simulink model "RAM_Design"  (R2025a)
settings: Solver=FixedStepDiscrete  StartTime=0.0  StopTime=10  FixedStep=1e-6  RelTol=1e-3
undefined symbols (not defined in the file): Bit_1, Bit_2, Bit_3, Bit_4, Bit_5, Bit_6, Bit_7, Bit_8
libraries: fl_lib x320, nesl_utility x136, simulink_extras x57
(part 3 of 5)

== system RAM_Design/Subsystem1/8Bit RAM 63/Subsystem13 ==
  Enable : Inport
  Data : Inport  Port=2
  Store : Inport  Port=3
  AND : Logic  IconShape=distinctive  AllPortsSameDT=off  OutDataTypeStr=boolean
  Cast To Double : DataTypeConversion  OutDataTypeStr=double  SaturateOnIntegerOverflow=off  RndMeth=Floor
  Controlled Voltage Source : fl_lib/Electrical/Electrical Sources/Controlled Voltage Source
  D Latch : simulink_extras/Flip Flops/D Latch
  Delay One Step : Delay  DelayLength=1
  Electrical Reference : fl_lib/Electrical/Electrical Elements/Electrical Reference
  Gain : Gain  Gain=5
  Simulink-PS Converter : nesl_utility/Simulink-PS Converter  PhysicalDomain=network_engine_domain  SubClassName=ps_input  LeftPortType=input  RightPortType=output  PseudoPeriodic=off  Frequencies=[]  NoiseDistribution=none  NoiseParameters=[]  Unit=1  AffineConversion=off  FilteringAndDerivatives=provide  SimscapeFilterOrder=1  InputFilterTimeConstant=0.001  UdotUserProvided=0
  Q : PMIOPort  Side=Right
  StoredVal : Outport
  wires:
  AND/1 -> Delay One Step/1
  Store/1 -> D Latch/2
  Gain/1 -> Simulink-PS Converter/1
  D Latch/1 -> StoredVal/1, AND/1
  Cast To Double/1 -> Gain/1
  Enable/1 -> AND/2
  Data/1 -> D Latch/1
  Delay One Step/1 -> Cast To Double/1
  connections:
  Controlled Voltage Source/RConn1 -- Simulink-PS Converter/RConn1
  Electrical Reference/LConn1 -- Controlled Voltage Source/RConn2
  Controlled Voltage Source/LConn1 -- Q/RConn1

== system RAM_Design/Subsystem1/8Bit RAM 63/Subsystem14 ==
  Enable : Inport
  Data : Inport  Port=2
  Store : Inport  Port=3
  AND : Logic  IconShape=distinctive  AllPortsSameDT=off  OutDataTypeStr=boolean
  Cast To Double : DataTypeConversion  OutDataTypeStr=double  SaturateOnIntegerOverflow=off  RndMeth=Floor
  Controlled Voltage Source : fl_lib/Electrical/Electrical Sources/Controlled Voltage Source
  D Latch : simulink_extras/Flip Flops/D Latch
  Delay One Step : Delay  DelayLength=1
  Electrical Reference : fl_lib/Electrical/Electrical Elements/Electrical Reference
  Gain : Gain  Gain=5
  Simulink-PS Converter : nesl_utility/Simulink-PS Converter  PhysicalDomain=network_engine_domain  SubClassName=ps_input  LeftPortType=input  RightPortType=output  PseudoPeriodic=off  Frequencies=[]  NoiseDistribution=none  NoiseParameters=[]  Unit=1  AffineConversion=off  FilteringAndDerivatives=provide  SimscapeFilterOrder=1  InputFilterTimeConstant=0.001  UdotUserProvided=0
  Q : PMIOPort  Side=Right
  StoredVal : Outport
  wires:
  AND/1 -> Delay One Step/1
  Store/1 -> D Latch/2
  Gain/1 -> Simulink-PS Converter/1
  D Latch/1 -> StoredVal/1, AND/1
  Cast To Double/1 -> Gain/1
  Enable/1 -> AND/2
  Data/1 -> D Latch/1
  Delay One Step/1 -> Cast To Double/1
  connections:
  Controlled Voltage Source/RConn1 -- Simulink-PS Converter/RConn1
  Electrical Reference/LConn1 -- Controlled Voltage Source/RConn2
  Controlled Voltage Source/LConn1 -- Q/RConn1

== system RAM_Design/Subsystem1/8Bit RAM 63/Subsystem15 ==
  Enable : Inport
  Data : Inport  Port=2
  Store : Inport  Port=3
  AND : Logic  IconShape=distinctive  AllPortsSameDT=off  OutDataTypeStr=boolean
  Cast To Double : DataTypeConversion  OutDataTypeStr=double  SaturateOnIntegerOverflow=off  RndMeth=Floor
  Controlled Voltage Source : fl_lib/Electrical/Electrical Sources/Controlled Voltage Source
  D Latch : simulink_extras/Flip Flops/D Latch
  Delay One Step : Delay  DelayLength=1
  Electrical Reference : fl_lib/Electrical/Electrical Elements/Electrical Reference
  Gain : Gain  Gain=5
  Simulink-PS Converter : nesl_utility/Simulink-PS Converter  PhysicalDomain=network_engine_domain  SubClassName=ps_input  LeftPortType=input  RightPortType=output  PseudoPeriodic=off  Frequencies=[]  NoiseDistribution=none  NoiseParameters=[]  Unit=1  AffineConversion=off  FilteringAndDerivatives=provide  SimscapeFilterOrder=1  InputFilterTimeConstant=0.001  UdotUserProvided=0
  Q : PMIOPort  Side=Right
  StoredVal : Outport
  wires:
  AND/1 -> Delay One Step/1
  Store/1 -> D Latch/2
  Gain/1 -> Simulink-PS Converter/1
  D Latch/1 -> StoredVal/1, AND/1
  Cast To Double/1 -> Gain/1
  Enable/1 -> AND/2
  Data/1 -> D Latch/1
  Delay One Step/1 -> Cast To Double/1
  connections:
  Controlled Voltage Source/RConn1 -- Simulink-PS Converter/RConn1
  Electrical Reference/LConn1 -- Controlled Voltage Source/RConn2
  Controlled Voltage Source/LConn1 -- Q/RConn1

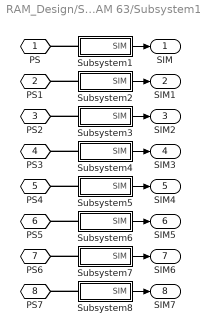
== system RAM_Design/Subsystem1/8Bit RAM 63/Subsystem16 ==
  Subsystem1 : Subsystem
  Subsystem2 : Subsystem
  Subsystem3 : Subsystem
  Subsystem4 : Subsystem
  Subsystem5 : Subsystem
  Subsystem6 : Subsystem
  Subsystem7 : Subsystem
  Subsystem8 : Subsystem
  PS : PMIOPort  Side=Left
  PS1 : PMIOPort  Port=2  Side=Left
  PS2 : PMIOPort  Port=3  Side=Left
  PS3 : PMIOPort  Port=4  Side=Left
  PS4 : PMIOPort  Port=5  Side=Left
  PS5 : PMIOPort  Port=6  Side=Left
  PS6 : PMIOPort  Port=7  Side=Left
  PS7 : PMIOPort  Port=8  Side=Left
  SIM : Outport
  SIM1 : Outport  Port=2
  SIM2 : Outport  Port=3
  SIM3 : Outport  Port=4
  SIM4 : Outport  Port=5
  SIM5 : Outport  Port=6
  SIM6 : Outport  Port=7
  SIM7 : Outport  Port=8
  wires:
  Subsystem7/1(SIM) -> SIM6/1
  Subsystem8/1(SIM) -> SIM7/1
  Subsystem3/1(SIM) -> SIM2/1
  Subsystem4/1(SIM) -> SIM3/1
  Subsystem6/1(SIM) -> SIM5/1
  Subsystem2/1(SIM) -> SIM1/1
  Subsystem5/1(SIM) -> SIM4/1
  Subsystem1/1(SIM) -> SIM/1
  connections:
  Subsystem1/LConn1 -- PS/RConn1
  Subsystem8/LConn1 -- PS7/RConn1
  Subsystem5/LConn1 -- PS4/RConn1
  Subsystem6/LConn1 -- PS5/RConn1
  Subsystem7/LConn1 -- PS6/RConn1
  Subsystem3/LConn1 -- PS2/RConn1
  Subsystem4/LConn1 -- PS3/RConn1
  Subsystem2/LConn1 -- PS1/RConn1

== system RAM_Design/Subsystem1/8Bit RAM 63/Subsystem2 ==
  Cast To Boolean : DataTypeConversion  OutDataTypeStr=boolean  SaturateOnIntegerOverflow=off  RndMeth=Floor
  Delay One Step : Delay  DelayLength=1
  Electrical Reference : fl_lib/Electrical/Electrical Elements/Electrical Reference
  Gain : Gain  Gain=0.2
  PS-Simulink Converter : nesl_utility/PS-Simulink Converter  PhysicalDomain=network_engine_domain  SubClassName=ps_output  LeftPortType=input  RightPortType=output  PseudoPeriodic=off  Frequencies=[]  VectorFormat=inherit  Unit=inherit  AffineConversion=off
  Voltage Sensor : fl_lib/Electrical/Electrical Sensors/Voltage Sensor
  PS : PMIOPort  Side=Left
  SIM : Outport
  wires:
  PS-Simulink Converter/1 -> Gain/1
  Cast To Boolean/1 -> Delay One Step/1
  Gain/1 -> Cast To Boolean/1
  Delay One Step/1 -> SIM/1
  connections:
  PS/RConn1 -- Voltage Sensor/LConn1
  Electrical Reference/LConn1 -- Voltage Sensor/RConn2
  PS-Simulink Converter/LConn1 -- Voltage Sensor/RConn1

== system RAM_Design/Subsystem1/8Bit RAM 63/Subsystem3 ==
  Cast To Boolean : DataTypeConversion  OutDataTypeStr=boolean  SaturateOnIntegerOverflow=off  RndMeth=Floor
  Delay One Step : Delay  DelayLength=1
  Electrical Reference : fl_lib/Electrical/Electrical Elements/Electrical Reference
  Gain : Gain  Gain=0.2
  PS-Simulink Converter : nesl_utility/PS-Simulink Converter  PhysicalDomain=network_engine_domain  SubClassName=ps_output  LeftPortType=input  RightPortType=output  PseudoPeriodic=off  Frequencies=[]  VectorFormat=inherit  Unit=inherit  AffineConversion=off
  Voltage Sensor : fl_lib/Electrical/Electrical Sensors/Voltage Sensor
  PS : PMIOPort  Side=Left
  SIM : Outport
  wires:
  PS-Simulink Converter/1 -> Gain/1
  Cast To Boolean/1 -> Delay One Step/1
  Gain/1 -> Cast To Boolean/1
  Delay One Step/1 -> SIM/1
  connections:
  PS/RConn1 -- Voltage Sensor/LConn1
  Electrical Reference/LConn1 -- Voltage Sensor/RConn2
  PS-Simulink Converter/LConn1 -- Voltage Sensor/RConn1

== system RAM_Design/Subsystem1/8Bit RAM 63/Subsystem4 ==
  Cast To Boolean : DataTypeConversion  OutDataTypeStr=boolean  SaturateOnIntegerOverflow=off  RndMeth=Floor
  Delay One Step : Delay  DelayLength=1
  Electrical Reference : fl_lib/Electrical/Electrical Elements/Electrical Reference
  Gain : Gain  Gain=0.2
  PS-Simulink Converter : nesl_utility/PS-Simulink Converter  PhysicalDomain=network_engine_domain  SubClassName=ps_output  LeftPortType=input  RightPortType=output  PseudoPeriodic=off  Frequencies=[]  VectorFormat=inherit  Unit=inherit  AffineConversion=off
  Voltage Sensor : fl_lib/Electrical/Electrical Sensors/Voltage Sensor
  PS : PMIOPort  Side=Left
  SIM : Outport
  wires:
  PS-Simulink Converter/1 -> Gain/1
  Cast To Boolean/1 -> Delay One Step/1
  Gain/1 -> Cast To Boolean/1
  Delay One Step/1 -> SIM/1
  connections:
  PS/RConn1 -- Voltage Sensor/LConn1
  Electrical Reference/LConn1 -- Voltage Sensor/RConn2
  PS-Simulink Converter/LConn1 -- Voltage Sensor/RConn1

== system RAM_Design/Subsystem1/8Bit RAM 63/Subsystem5 ==
  Cast To Boolean : DataTypeConversion  OutDataTypeStr=boolean  SaturateOnIntegerOverflow=off  RndMeth=Floor
  Delay One Step : Delay  DelayLength=1
  Electrical Reference : fl_lib/Electrical/Electrical Elements/Electrical Reference
  Gain : Gain  Gain=0.2
  PS-Simulink Converter : nesl_utility/PS-Simulink Converter  PhysicalDomain=network_engine_domain  SubClassName=ps_output  LeftPortType=input  RightPortType=output  PseudoPeriodic=off  Frequencies=[]  VectorFormat=inherit  Unit=inherit  AffineConversion=off
  Voltage Sensor : fl_lib/Electrical/Electrical Sensors/Voltage Sensor
  PS : PMIOPort  Side=Left
  SIM : Outport
  wires:
  PS-Simulink Converter/1 -> Gain/1
  Cast To Boolean/1 -> Delay One Step/1
  Gain/1 -> Cast To Boolean/1
  Delay One Step/1 -> SIM/1
  connections:
  PS/RConn1 -- Voltage Sensor/LConn1
  Electrical Reference/LConn1 -- Voltage Sensor/RConn2
  PS-Simulink Converter/LConn1 -- Voltage Sensor/RConn1

== system RAM_Design/Subsystem1/8Bit RAM 63/Subsystem6 ==
  Cast To Boolean : DataTypeConversion  OutDataTypeStr=boolean  SaturateOnIntegerOverflow=off  RndMeth=Floor
  Delay One Step : Delay  DelayLength=1
  Electrical Reference : fl_lib/Electrical/Electrical Elements/Electrical Reference
  Gain : Gain  Gain=0.2
  PS-Simulink Converter : nesl_utility/PS-Simulink Converter  PhysicalDomain=network_engine_domain  SubClassName=ps_output  LeftPortType=input  RightPortType=output  PseudoPeriodic=off  Frequencies=[]  VectorFormat=inherit  Unit=inherit  AffineConversion=off
  Voltage Sensor : fl_lib/Electrical/Electrical Sensors/Voltage Sensor
  PS : PMIOPort  Side=Left
  SIM : Outport
  wires:
  PS-Simulink Converter/1 -> Gain/1
  Cast To Boolean/1 -> Delay One Step/1
  Gain/1 -> Cast To Boolean/1
  Delay One Step/1 -> SIM/1
  connections:
  PS/RConn1 -- Voltage Sensor/LConn1
  Electrical Reference/LConn1 -- Voltage Sensor/RConn2
  PS-Simulink Converter/LConn1 -- Voltage Sensor/RConn1

== system RAM_Design/Subsystem1/8Bit RAM 63/Subsystem7 ==
  Cast To Boolean : DataTypeConversion  OutDataTypeStr=boolean  SaturateOnIntegerOverflow=off  RndMeth=Floor
  Delay One Step : Delay  DelayLength=1
  Electrical Reference : fl_lib/Electrical/Electrical Elements/Electrical Reference
  Gain : Gain  Gain=0.2
  PS-Simulink Converter : nesl_utility/PS-Simulink Converter  PhysicalDomain=network_engine_domain  SubClassName=ps_output  LeftPortType=input  RightPortType=output  PseudoPeriodic=off  Frequencies=[]  VectorFormat=inherit  Unit=inherit  AffineConversion=off
  Voltage Sensor : fl_lib/Electrical/Electrical Sensors/Voltage Sensor
  PS : PMIOPort  Side=Left
  SIM : Outport
  wires:
  PS-Simulink Converter/1 -> Gain/1
  Cast To Boolean/1 -> Delay One Step/1
  Gain/1 -> Cast To Boolean/1
  Delay One Step/1 -> SIM/1
  connections:
  PS/RConn1 -- Voltage Sensor/LConn1
  Electrical Reference/LConn1 -- Voltage Sensor/RConn2
  PS-Simulink Converter/LConn1 -- Voltage Sensor/RConn1

== system RAM_Design/Subsystem1/8Bit RAM 63/Subsystem8 ==
  Cast To Boolean : DataTypeConversion  OutDataTypeStr=boolean  SaturateOnIntegerOverflow=off  RndMeth=Floor
  Delay One Step : Delay  DelayLength=1
  Electrical Reference : fl_lib/Electrical/Electrical Elements/Electrical Reference
  Gain : Gain  Gain=0.2
  PS-Simulink Converter : nesl_utility/PS-Simulink Converter  PhysicalDomain=network_engine_domain  SubClassName=ps_output  LeftPortType=input  RightPortType=output  PseudoPeriodic=off  Frequencies=[]  VectorFormat=inherit  Unit=inherit  AffineConversion=off
  Voltage Sensor : fl_lib/Electrical/Electrical Sensors/Voltage Sensor
  PS : PMIOPort  Side=Left
  SIM : Outport
  wires:
  PS-Simulink Converter/1 -> Gain/1
  Cast To Boolean/1 -> Delay One Step/1
  Gain/1 -> Cast To Boolean/1
  Delay One Step/1 -> SIM/1
  connections:
  PS/RConn1 -- Voltage Sensor/LConn1
  Electrical Reference/LConn1 -- Voltage Sensor/RConn2
  PS-Simulink Converter/LConn1 -- Voltage Sensor/RConn1

== system RAM_Design/Subsystem1/8Bit RAM 63/Subsystem9 ==
  Enable : Inport
  Data : Inport  Port=2
  Store : Inport  Port=3
  AND : Logic  IconShape=distinctive  AllPortsSameDT=off  OutDataTypeStr=boolean
  Cast To Double : DataTypeConversion  OutDataTypeStr=double  SaturateOnIntegerOverflow=off  RndMeth=Floor
  Controlled Voltage Source : fl_lib/Electrical/Electrical Sources/Controlled Voltage Source
  D Latch : simulink_extras/Flip Flops/D Latch
  Delay One Step : Delay  DelayLength=1
  Electrical Reference : fl_lib/Electrical/Electrical Elements/Electrical Reference
  Gain : Gain  Gain=5
  Simulink-PS Converter : nesl_utility/Simulink-PS Converter  PhysicalDomain=network_engine_domain  SubClassName=ps_input  LeftPortType=input  RightPortType=output  PseudoPeriodic=off  Frequencies=[]  NoiseDistribution=none  NoiseParameters=[]  Unit=1  AffineConversion=off  FilteringAndDerivatives=provide  SimscapeFilterOrder=1  InputFilterTimeConstant=0.001  UdotUserProvided=0
  Q : PMIOPort  Side=Right
  StoredVal : Outport
  wires:
  AND/1 -> Delay One Step/1
  Store/1 -> D Latch/2
  Gain/1 -> Simulink-PS Converter/1
  D Latch/1 -> StoredVal/1, AND/1
  Cast To Double/1 -> Gain/1
  Enable/1 -> AND/2
  Data/1 -> D Latch/1
  Delay One Step/1 -> Cast To Double/1
  connections:
  Controlled Voltage Source/RConn1 -- Simulink-PS Converter/RConn1
  Electrical Reference/LConn1 -- Controlled Voltage Source/RConn2
  Controlled Voltage Source/LConn1 -- Q/RConn1

== system RAM_Design/Subsystem1/8Bit RAM 7/Subsystem ==
  Cast To Boolean : DataTypeConversion  OutDataTypeStr=boolean  SaturateOnIntegerOverflow=off  RndMeth=Floor
  Delay One Step : Delay  DelayLength=1
  Electrical Reference : fl_lib/Electrical/Electrical Elements/Electrical Reference
  Gain : Gain  Gain=0.2
  PS-Simulink Converter : nesl_utility/PS-Simulink Converter  PhysicalDomain=network_engine_domain  SubClassName=ps_output  LeftPortType=input  RightPortType=output  PseudoPeriodic=off  Frequencies=[]  VectorFormat=inherit  Unit=inherit  AffineConversion=off
  Voltage Sensor : fl_lib/Electrical/Electrical Sensors/Voltage Sensor
  PS : PMIOPort  Side=Left
  SIM : Outport
  wires:
  PS-Simulink Converter/1 -> Gain/1
  Cast To Boolean/1 -> Delay One Step/1
  Gain/1 -> Cast To Boolean/1
  Delay One Step/1 -> SIM/1
  connections:
  PS/RConn1 -- Voltage Sensor/LConn1
  Electrical Reference/LConn1 -- Voltage Sensor/RConn2
  PS-Simulink Converter/LConn1 -- Voltage Sensor/RConn1

== system RAM_Design/Subsystem1/8Bit RAM 7/Subsystem1 ==
  Enable : Inport
  Data : Inport  Port=2
  Store : Inport  Port=3
  AND : Logic  IconShape=distinctive  AllPortsSameDT=off  OutDataTypeStr=boolean
  Cast To Double : DataTypeConversion  OutDataTypeStr=double  SaturateOnIntegerOverflow=off  RndMeth=Floor
  Controlled Voltage Source : fl_lib/Electrical/Electrical Sources/Controlled Voltage Source
  D Latch : simulink_extras/Flip Flops/D Latch
  Delay One Step : Delay  DelayLength=1
  Electrical Reference : fl_lib/Electrical/Electrical Elements/Electrical Reference
  Gain : Gain  Gain=5
  Simulink-PS Converter : nesl_utility/Simulink-PS Converter  PhysicalDomain=network_engine_domain  SubClassName=ps_input  LeftPortType=input  RightPortType=output  PseudoPeriodic=off  Frequencies=[]  NoiseDistribution=none  NoiseParameters=[]  Unit=1  AffineConversion=off  FilteringAndDerivatives=provide  SimscapeFilterOrder=1  InputFilterTimeConstant=0.001  UdotUserProvided=0
  Q : PMIOPort  Side=Right
  StoredVal : Outport
  wires:
  AND/1 -> Delay One Step/1
  Store/1 -> D Latch/2
  Gain/1 -> Simulink-PS Converter/1
  D Latch/1 -> StoredVal/1, AND/1
  Cast To Double/1 -> Gain/1
  Enable/1 -> AND/2
  Data/1 -> D Latch/1
  Delay One Step/1 -> Cast To Double/1
  connections:
  Controlled Voltage Source/RConn1 -- Simulink-PS Converter/RConn1
  Electrical Reference/LConn1 -- Controlled Voltage Source/RConn2
  Controlled Voltage Source/LConn1 -- Q/RConn1

== system RAM_Design/Subsystem1/8Bit RAM 7/Subsystem10 ==
  Enable : Inport
  Data : Inport  Port=2
  Store : Inport  Port=3
  AND : Logic  IconShape=distinctive  AllPortsSameDT=off  OutDataTypeStr=boolean
  Cast To Double : DataTypeConversion  OutDataTypeStr=double  SaturateOnIntegerOverflow=off  RndMeth=Floor
  Controlled Voltage Source : fl_lib/Electrical/Electrical Sources/Controlled Voltage Source
  D Latch : simulink_extras/Flip Flops/D Latch
  Delay One Step : Delay  DelayLength=1
  Electrical Reference : fl_lib/Electrical/Electrical Elements/Electrical Reference
  Gain : Gain  Gain=5
  Simulink-PS Converter : nesl_utility/Simulink-PS Converter  PhysicalDomain=network_engine_domain  SubClassName=ps_input  LeftPortType=input  RightPortType=output  PseudoPeriodic=off  Frequencies=[]  NoiseDistribution=none  NoiseParameters=[]  Unit=1  AffineConversion=off  FilteringAndDerivatives=provide  SimscapeFilterOrder=1  InputFilterTimeConstant=0.001  UdotUserProvided=0
  Q : PMIOPort  Side=Right
  StoredVal : Outport
  wires:
  AND/1 -> Delay One Step/1
  Store/1 -> D Latch/2
  Gain/1 -> Simulink-PS Converter/1
  D Latch/1 -> StoredVal/1, AND/1
  Cast To Double/1 -> Gain/1
  Enable/1 -> AND/2
  Data/1 -> D Latch/1
  Delay One Step/1 -> Cast To Double/1
  connections:
  Controlled Voltage Source/RConn1 -- Simulink-PS Converter/RConn1
  Electrical Reference/LConn1 -- Controlled Voltage Source/RConn2
  Controlled Voltage Source/LConn1 -- Q/RConn1

== system RAM_Design/Subsystem1/8Bit RAM 7/Subsystem11 ==
  Enable : Inport
  Data : Inport  Port=2
  Store : Inport  Port=3
  AND : Logic  IconShape=distinctive  AllPortsSameDT=off  OutDataTypeStr=boolean
  Cast To Double : DataTypeConversion  OutDataTypeStr=double  SaturateOnIntegerOverflow=off  RndMeth=Floor
  Controlled Voltage Source : fl_lib/Electrical/Electrical Sources/Controlled Voltage Source
  D Latch : simulink_extras/Flip Flops/D Latch
  Delay One Step : Delay  DelayLength=1
  Electrical Reference : fl_lib/Electrical/Electrical Elements/Electrical Reference
  Gain : Gain  Gain=5
  Simulink-PS Converter : nesl_utility/Simulink-PS Converter  PhysicalDomain=network_engine_domain  SubClassName=ps_input  LeftPortType=input  RightPortType=output  PseudoPeriodic=off  Frequencies=[]  NoiseDistribution=none  NoiseParameters=[]  Unit=1  AffineConversion=off  FilteringAndDerivatives=provide  SimscapeFilterOrder=1  InputFilterTimeConstant=0.001  UdotUserProvided=0
  Q : PMIOPort  Side=Right
  StoredVal : Outport
  wires:
  AND/1 -> Delay One Step/1
  Store/1 -> D Latch/2
  Gain/1 -> Simulink-PS Converter/1
  D Latch/1 -> StoredVal/1, AND/1
  Cast To Double/1 -> Gain/1
  Enable/1 -> AND/2
  Data/1 -> D Latch/1
  Delay One Step/1 -> Cast To Double/1
  connections:
  Controlled Voltage Source/RConn1 -- Simulink-PS Converter/RConn1
  Electrical Reference/LConn1 -- Controlled Voltage Source/RConn2
  Controlled Voltage Source/LConn1 -- Q/RConn1

== system RAM_Design/Subsystem1/8Bit RAM 7/Subsystem12 ==
  Enable : Inport
  Data : Inport  Port=2
  Store : Inport  Port=3
  AND : Logic  IconShape=distinctive  AllPortsSameDT=off  OutDataTypeStr=boolean
  Cast To Double : DataTypeConversion  OutDataTypeStr=double  SaturateOnIntegerOverflow=off  RndMeth=Floor
  Controlled Voltage Source : fl_lib/Electrical/Electrical Sources/Controlled Voltage Source
  D Latch : simulink_extras/Flip Flops/D Latch
  Delay One Step : Delay  DelayLength=1
  Electrical Reference : fl_lib/Electrical/Electrical Elements/Electrical Reference
  Gain : Gain  Gain=5
  Simulink-PS Converter : nesl_utility/Simulink-PS Converter  PhysicalDomain=network_engine_domain  SubClassName=ps_input  LeftPortType=input  RightPortType=output  PseudoPeriodic=off  Frequencies=[]  NoiseDistribution=none  NoiseParameters=[]  Unit=1  AffineConversion=off  FilteringAndDerivatives=provide  SimscapeFilterOrder=1  InputFilterTimeConstant=0.001  UdotUserProvided=0
  Q : PMIOPort  Side=Right
  StoredVal : Outport
  wires:
  AND/1 -> Delay One Step/1
  Store/1 -> D Latch/2
  Gain/1 -> Simulink-PS Converter/1
  D Latch/1 -> StoredVal/1, AND/1
  Cast To Double/1 -> Gain/1
  Enable/1 -> AND/2
  Data/1 -> D Latch/1
  Delay One Step/1 -> Cast To Double/1
  connections:
  Controlled Voltage Source/RConn1 -- Simulink-PS Converter/RConn1
  Electrical Reference/LConn1 -- Controlled Voltage Source/RConn2
  Controlled Voltage Source/LConn1 -- Q/RConn1

== system RAM_Design/Subsystem1/8Bit RAM 7/Subsystem13 ==
  Enable : Inport
  Data : Inport  Port=2
  Store : Inport  Port=3
  AND : Logic  IconShape=distinctive  AllPortsSameDT=off  OutDataTypeStr=boolean
  Cast To Double : DataTypeConversion  OutDataTypeStr=double  SaturateOnIntegerOverflow=off  RndMeth=Floor
  Controlled Voltage Source : fl_lib/Electrical/Electrical Sources/Controlled Voltage Source
  D Latch : simulink_extras/Flip Flops/D Latch
  Delay One Step : Delay  DelayLength=1
  Electrical Reference : fl_lib/Electrical/Electrical Elements/Electrical Reference
  Gain : Gain  Gain=5
  Simulink-PS Converter : nesl_utility/Simulink-PS Converter  PhysicalDomain=network_engine_domain  SubClassName=ps_input  LeftPortType=input  RightPortType=output  PseudoPeriodic=off  Frequencies=[]  NoiseDistribution=none  NoiseParameters=[]  Unit=1  AffineConversion=off  FilteringAndDerivatives=provide  SimscapeFilterOrder=1  InputFilterTimeConstant=0.001  UdotUserProvided=0
  Q : PMIOPort  Side=Right
  StoredVal : Outport
  wires:
  AND/1 -> Delay One Step/1
  Store/1 -> D Latch/2
  Gain/1 -> Simulink-PS Converter/1
  D Latch/1 -> StoredVal/1, AND/1
  Cast To Double/1 -> Gain/1
  Enable/1 -> AND/2
  Data/1 -> D Latch/1
  Delay One Step/1 -> Cast To Double/1
  connections:
  Controlled Voltage Source/RConn1 -- Simulink-PS Converter/RConn1
  Electrical Reference/LConn1 -- Controlled Voltage Source/RConn2
  Controlled Voltage Source/LConn1 -- Q/RConn1

== system RAM_Design/Subsystem1/8Bit RAM 7/Subsystem14 ==
  Enable : Inport
  Data : Inport  Port=2
  Store : Inport  Port=3
  AND : Logic  IconShape=distinctive  AllPortsSameDT=off  OutDataTypeStr=boolean
  Cast To Double : DataTypeConversion  OutDataTypeStr=double  SaturateOnIntegerOverflow=off  RndMeth=Floor
  Controlled Voltage Source : fl_lib/Electrical/Electrical Sources/Controlled Voltage Source
  D Latch : simulink_extras/Flip Flops/D Latch
  Delay One Step : Delay  DelayLength=1
  Electrical Reference : fl_lib/Electrical/Electrical Elements/Electrical Reference
  Gain : Gain  Gain=5
  Simulink-PS Converter : nesl_utility/Simulink-PS Converter  PhysicalDomain=network_engine_domain  SubClassName=ps_input  LeftPortType=input  RightPortType=output  PseudoPeriodic=off  Frequencies=[]  NoiseDistribution=none  NoiseParameters=[]  Unit=1  AffineConversion=off  FilteringAndDerivatives=provide  SimscapeFilterOrder=1  InputFilterTimeConstant=0.001  UdotUserProvided=0
  Q : PMIOPort  Side=Right
  StoredVal : Outport
  wires:
  AND/1 -> Delay One Step/1
  Store/1 -> D Latch/2
  Gain/1 -> Simulink-PS Converter/1
  D Latch/1 -> StoredVal/1, AND/1
  Cast To Double/1 -> Gain/1
  Enable/1 -> AND/2
  Data/1 -> D Latch/1
  Delay One Step/1 -> Cast To Double/1
  connections:
  Controlled Voltage Source/RConn1 -- Simulink-PS Converter/RConn1
  Electrical Reference/LConn1 -- Controlled Voltage Source/RConn2
  Controlled Voltage Source/LConn1 -- Q/RConn1

== system RAM_Design/Subsystem1/8Bit RAM 7/Subsystem15 ==
  Enable : Inport
  Data : Inport  Port=2
  Store : Inport  Port=3
  AND : Logic  IconShape=distinctive  AllPortsSameDT=off  OutDataTypeStr=boolean
  Cast To Double : DataTypeConversion  OutDataTypeStr=double  SaturateOnIntegerOverflow=off  RndMeth=Floor
  Controlled Voltage Source : fl_lib/Electrical/Electrical Sources/Controlled Voltage Source
  D Latch : simulink_extras/Flip Flops/D Latch
  Delay One Step : Delay  DelayLength=1
  Electrical Reference : fl_lib/Electrical/Electrical Elements/Electrical Reference
  Gain : Gain  Gain=5
  Simulink-PS Converter : nesl_utility/Simulink-PS Converter  PhysicalDomain=network_engine_domain  SubClassName=ps_input  LeftPortType=input  RightPortType=output  PseudoPeriodic=off  Frequencies=[]  NoiseDistribution=none  NoiseParameters=[]  Unit=1  AffineConversion=off  FilteringAndDerivatives=provide  SimscapeFilterOrder=1  InputFilterTimeConstant=0.001  UdotUserProvided=0
  Q : PMIOPort  Side=Right
  StoredVal : Outport
  wires:
  AND/1 -> Delay One Step/1
  Store/1 -> D Latch/2
  Gain/1 -> Simulink-PS Converter/1
  D Latch/1 -> StoredVal/1, AND/1
  Cast To Double/1 -> Gain/1
  Enable/1 -> AND/2
  Data/1 -> D Latch/1
  Delay One Step/1 -> Cast To Double/1
  connections:
  Controlled Voltage Source/RConn1 -- Simulink-PS Converter/RConn1
  Electrical Reference/LConn1 -- Controlled Voltage Source/RConn2
  Controlled Voltage Source/LConn1 -- Q/RConn1

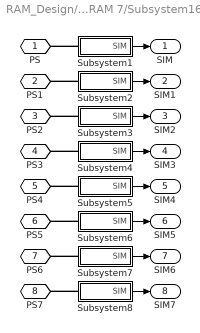
== system RAM_Design/Subsystem1/8Bit RAM 7/Subsystem16 ==
  Subsystem1 : Subsystem
  Subsystem2 : Subsystem
  Subsystem3 : Subsystem
  Subsystem4 : Subsystem
  Subsystem5 : Subsystem
  Subsystem6 : Subsystem
  Subsystem7 : Subsystem
  Subsystem8 : Subsystem
  PS : PMIOPort  Side=Left
  PS1 : PMIOPort  Port=2  Side=Left
  PS2 : PMIOPort  Port=3  Side=Left
  PS3 : PMIOPort  Port=4  Side=Left
  PS4 : PMIOPort  Port=5  Side=Left
  PS5 : PMIOPort  Port=6  Side=Left
  PS6 : PMIOPort  Port=7  Side=Left
  PS7 : PMIOPort  Port=8  Side=Left
  SIM : Outport
  SIM1 : Outport  Port=2
  SIM2 : Outport  Port=3
  SIM3 : Outport  Port=4
  SIM4 : Outport  Port=5
  SIM5 : Outport  Port=6
  SIM6 : Outport  Port=7
  SIM7 : Outport  Port=8
  wires:
  Subsystem7/1(SIM) -> SIM6/1
  Subsystem8/1(SIM) -> SIM7/1
  Subsystem3/1(SIM) -> SIM2/1
  Subsystem4/1(SIM) -> SIM3/1
  Subsystem6/1(SIM) -> SIM5/1
  Subsystem2/1(SIM) -> SIM1/1
  Subsystem5/1(SIM) -> SIM4/1
  Subsystem1/1(SIM) -> SIM/1
  connections:
  Subsystem1/LConn1 -- PS/RConn1
  Subsystem8/LConn1 -- PS7/RConn1
  Subsystem5/LConn1 -- PS4/RConn1
  Subsystem6/LConn1 -- PS5/RConn1
  Subsystem7/LConn1 -- PS6/RConn1
  Subsystem3/LConn1 -- PS2/RConn1
  Subsystem4/LConn1 -- PS3/RConn1
  Subsystem2/LConn1 -- PS1/RConn1

== system RAM_Design/Subsystem1/8Bit RAM 7/Subsystem2 ==
  Cast To Boolean : DataTypeConversion  OutDataTypeStr=boolean  SaturateOnIntegerOverflow=off  RndMeth=Floor
  Delay One Step : Delay  DelayLength=1
  Electrical Reference : fl_lib/Electrical/Electrical Elements/Electrical Reference
  Gain : Gain  Gain=0.2
  PS-Simulink Converter : nesl_utility/PS-Simulink Converter  PhysicalDomain=network_engine_domain  SubClassName=ps_output  LeftPortType=input  RightPortType=output  PseudoPeriodic=off  Frequencies=[]  VectorFormat=inherit  Unit=inherit  AffineConversion=off
  Voltage Sensor : fl_lib/Electrical/Electrical Sensors/Voltage Sensor
  PS : PMIOPort  Side=Left
  SIM : Outport
  wires:
  PS-Simulink Converter/1 -> Gain/1
  Cast To Boolean/1 -> Delay One Step/1
  Gain/1 -> Cast To Boolean/1
  Delay One Step/1 -> SIM/1
  connections:
  PS/RConn1 -- Voltage Sensor/LConn1
  Electrical Reference/LConn1 -- Voltage Sensor/RConn2
  PS-Simulink Converter/LConn1 -- Voltage Sensor/RConn1

== system RAM_Design/Subsystem1/8Bit RAM 7/Subsystem3 ==
  Cast To Boolean : DataTypeConversion  OutDataTypeStr=boolean  SaturateOnIntegerOverflow=off  RndMeth=Floor
  Delay One Step : Delay  DelayLength=1
  Electrical Reference : fl_lib/Electrical/Electrical Elements/Electrical Reference
  Gain : Gain  Gain=0.2
  PS-Simulink Converter : nesl_utility/PS-Simulink Converter  PhysicalDomain=network_engine_domain  SubClassName=ps_output  LeftPortType=input  RightPortType=output  PseudoPeriodic=off  Frequencies=[]  VectorFormat=inherit  Unit=inherit  AffineConversion=off
  Voltage Sensor : fl_lib/Electrical/Electrical Sensors/Voltage Sensor
  PS : PMIOPort  Side=Left
  SIM : Outport
  wires:
  PS-Simulink Converter/1 -> Gain/1
  Cast To Boolean/1 -> Delay One Step/1
  Gain/1 -> Cast To Boolean/1
  Delay One Step/1 -> SIM/1
  connections:
  PS/RConn1 -- Voltage Sensor/LConn1
  Electrical Reference/LConn1 -- Voltage Sensor/RConn2
  PS-Simulink Converter/LConn1 -- Voltage Sensor/RConn1

== system RAM_Design/Subsystem1/8Bit RAM 7/Subsystem4 ==
  Cast To Boolean : DataTypeConversion  OutDataTypeStr=boolean  SaturateOnIntegerOverflow=off  RndMeth=Floor
  Delay One Step : Delay  DelayLength=1
  Electrical Reference : fl_lib/Electrical/Electrical Elements/Electrical Reference
  Gain : Gain  Gain=0.2
  PS-Simulink Converter : nesl_utility/PS-Simulink Converter  PhysicalDomain=network_engine_domain  SubClassName=ps_output  LeftPortType=input  RightPortType=output  PseudoPeriodic=off  Frequencies=[]  VectorFormat=inherit  Unit=inherit  AffineConversion=off
  Voltage Sensor : fl_lib/Electrical/Electrical Sensors/Voltage Sensor
  PS : PMIOPort  Side=Left
  SIM : Outport
  wires:
  PS-Simulink Converter/1 -> Gain/1
  Cast To Boolean/1 -> Delay One Step/1
  Gain/1 -> Cast To Boolean/1
  Delay One Step/1 -> SIM/1
  connections:
  PS/RConn1 -- Voltage Sensor/LConn1
  Electrical Reference/LConn1 -- Voltage Sensor/RConn2
  PS-Simulink Converter/LConn1 -- Voltage Sensor/RConn1

== system RAM_Design/Subsystem1/8Bit RAM 7/Subsystem5 ==
  Cast To Boolean : DataTypeConversion  OutDataTypeStr=boolean  SaturateOnIntegerOverflow=off  RndMeth=Floor
  Delay One Step : Delay  DelayLength=1
  Electrical Reference : fl_lib/Electrical/Electrical Elements/Electrical Reference
  Gain : Gain  Gain=0.2
  PS-Simulink Converter : nesl_utility/PS-Simulink Converter  PhysicalDomain=network_engine_domain  SubClassName=ps_output  LeftPortType=input  RightPortType=output  PseudoPeriodic=off  Frequencies=[]  VectorFormat=inherit  Unit=inherit  AffineConversion=off
  Voltage Sensor : fl_lib/Electrical/Electrical Sensors/Voltage Sensor
  PS : PMIOPort  Side=Left
  SIM : Outport
  wires:
  PS-Simulink Converter/1 -> Gain/1
  Cast To Boolean/1 -> Delay One Step/1
  Gain/1 -> Cast To Boolean/1
  Delay One Step/1 -> SIM/1
  connections:
  PS/RConn1 -- Voltage Sensor/LConn1
  Electrical Reference/LConn1 -- Voltage Sensor/RConn2
  PS-Simulink Converter/LConn1 -- Voltage Sensor/RConn1

== system RAM_Design/Subsystem1/8Bit RAM 7/Subsystem6 ==
  Cast To Boolean : DataTypeConversion  OutDataTypeStr=boolean  SaturateOnIntegerOverflow=off  RndMeth=Floor
  Delay One Step : Delay  DelayLength=1
  Electrical Reference : fl_lib/Electrical/Electrical Elements/Electrical Reference
  Gain : Gain  Gain=0.2
  PS-Simulink Converter : nesl_utility/PS-Simulink Converter  PhysicalDomain=network_engine_domain  SubClassName=ps_output  LeftPortType=input  RightPortType=output  PseudoPeriodic=off  Frequencies=[]  VectorFormat=inherit  Unit=inherit  AffineConversion=off
  Voltage Sensor : fl_lib/Electrical/Electrical Sensors/Voltage Sensor
  PS : PMIOPort  Side=Left
  SIM : Outport
  wires:
  PS-Simulink Converter/1 -> Gain/1
  Cast To Boolean/1 -> Delay One Step/1
  Gain/1 -> Cast To Boolean/1
  Delay One Step/1 -> SIM/1
  connections:
  PS/RConn1 -- Voltage Sensor/LConn1
  Electrical Reference/LConn1 -- Voltage Sensor/RConn2
  PS-Simulink Converter/LConn1 -- Voltage Sensor/RConn1

== system RAM_Design/Subsystem1/8Bit RAM 7/Subsystem7 ==
  Cast To Boolean : DataTypeConversion  OutDataTypeStr=boolean  SaturateOnIntegerOverflow=off  RndMeth=Floor
  Delay One Step : Delay  DelayLength=1
  Electrical Reference : fl_lib/Electrical/Electrical Elements/Electrical Reference
  Gain : Gain  Gain=0.2
  PS-Simulink Converter : nesl_utility/PS-Simulink Converter  PhysicalDomain=network_engine_domain  SubClassName=ps_output  LeftPortType=input  RightPortType=output  PseudoPeriodic=off  Frequencies=[]  VectorFormat=inherit  Unit=inherit  AffineConversion=off
  Voltage Sensor : fl_lib/Electrical/Electrical Sensors/Voltage Sensor
  PS : PMIOPort  Side=Left
  SIM : Outport
  wires:
  PS-Simulink Converter/1 -> Gain/1
  Cast To Boolean/1 -> Delay One Step/1
  Gain/1 -> Cast To Boolean/1
  Delay One Step/1 -> SIM/1
  connections:
  PS/RConn1 -- Voltage Sensor/LConn1
  Electrical Reference/LConn1 -- Voltage Sensor/RConn2
  PS-Simulink Converter/LConn1 -- Voltage Sensor/RConn1

== system RAM_Design/Subsystem1/8Bit RAM 7/Subsystem8 ==
  Cast To Boolean : DataTypeConversion  OutDataTypeStr=boolean  SaturateOnIntegerOverflow=off  RndMeth=Floor
  Delay One Step : Delay  DelayLength=1
  Electrical Reference : fl_lib/Electrical/Electrical Elements/Electrical Reference
  Gain : Gain  Gain=0.2
  PS-Simulink Converter : nesl_utility/PS-Simulink Converter  PhysicalDomain=network_engine_domain  SubClassName=ps_output  LeftPortType=input  RightPortType=output  PseudoPeriodic=off  Frequencies=[]  VectorFormat=inherit  Unit=inherit  AffineConversion=off
  Voltage Sensor : fl_lib/Electrical/Electrical Sensors/Voltage Sensor
  PS : PMIOPort  Side=Left
  SIM : Outport
  wires:
  PS-Simulink Converter/1 -> Gain/1
  Cast To Boolean/1 -> Delay One Step/1
  Gain/1 -> Cast To Boolean/1
  Delay One Step/1 -> SIM/1
  connections:
  PS/RConn1 -- Voltage Sensor/LConn1
  Electrical Reference/LConn1 -- Voltage Sensor/RConn2
  PS-Simulink Converter/LConn1 -- Voltage Sensor/RConn1

== system RAM_Design/Subsystem1/8Bit RAM 7/Subsystem9 ==
  Enable : Inport
  Data : Inport  Port=2
  Store : Inport  Port=3
  AND : Logic  IconShape=distinctive  AllPortsSameDT=off  OutDataTypeStr=boolean
  Cast To Double : DataTypeConversion  OutDataTypeStr=double  SaturateOnIntegerOverflow=off  RndMeth=Floor
  Controlled Voltage Source : fl_lib/Electrical/Electrical Sources/Controlled Voltage Source
  D Latch : simulink_extras/Flip Flops/D Latch
  Delay One Step : Delay  DelayLength=1
  Electrical Reference : fl_lib/Electrical/Electrical Elements/Electrical Reference
  Gain : Gain  Gain=5
  Simulink-PS Converter : nesl_utility/Simulink-PS Converter  PhysicalDomain=network_engine_domain  SubClassName=ps_input  LeftPortType=input  RightPortType=output  PseudoPeriodic=off  Frequencies=[]  NoiseDistribution=none  NoiseParameters=[]  Unit=1  AffineConversion=off  FilteringAndDerivatives=provide  SimscapeFilterOrder=1  InputFilterTimeConstant=0.001  UdotUserProvided=0
  Q : PMIOPort  Side=Right
  StoredVal : Outport
  wires:
  AND/1 -> Delay One Step/1
  Store/1 -> D Latch/2
  Gain/1 -> Simulink-PS Converter/1
  D Latch/1 -> StoredVal/1, AND/1
  Cast To Double/1 -> Gain/1
  Enable/1 -> AND/2
  Data/1 -> D Latch/1
  Delay One Step/1 -> Cast To Double/1
  connections:
  Controlled Voltage Source/RConn1 -- Simulink-PS Converter/RConn1
  Electrical Reference/LConn1 -- Controlled Voltage Source/RConn2
  Controlled Voltage Source/LConn1 -- Q/RConn1

== system RAM_Design/Subsystem1/8Bit RAM 8/Subsystem ==
  Cast To Boolean : DataTypeConversion  OutDataTypeStr=boolean  SaturateOnIntegerOverflow=off  RndMeth=Floor
  Delay One Step : Delay  DelayLength=1
  Electrical Reference : fl_lib/Electrical/Electrical Elements/Electrical Reference
  Gain : Gain  Gain=0.2
  PS-Simulink Converter : nesl_utility/PS-Simulink Converter  PhysicalDomain=network_engine_domain  SubClassName=ps_output  LeftPortType=input  RightPortType=output  PseudoPeriodic=off  Frequencies=[]  VectorFormat=inherit  Unit=inherit  AffineConversion=off
  Voltage Sensor : fl_lib/Electrical/Electrical Sensors/Voltage Sensor
  PS : PMIOPort  Side=Left
  SIM : Outport
  wires:
  PS-Simulink Converter/1 -> Gain/1
  Cast To Boolean/1 -> Delay One Step/1
  Gain/1 -> Cast To Boolean/1
  Delay One Step/1 -> SIM/1
  connections:
  PS/RConn1 -- Voltage Sensor/LConn1
  Electrical Reference/LConn1 -- Voltage Sensor/RConn2
  PS-Simulink Converter/LConn1 -- Voltage Sensor/RConn1

== system RAM_Design/Subsystem1/8Bit RAM 8/Subsystem1 ==
  Enable : Inport
  Data : Inport  Port=2
  Store : Inport  Port=3
  AND : Logic  IconShape=distinctive  AllPortsSameDT=off  OutDataTypeStr=boolean
  Cast To Double : DataTypeConversion  OutDataTypeStr=double  SaturateOnIntegerOverflow=off  RndMeth=Floor
  Controlled Voltage Source : fl_lib/Electrical/Electrical Sources/Controlled Voltage Source
  D Latch : simulink_extras/Flip Flops/D Latch
  Delay One Step : Delay  DelayLength=1
  Electrical Reference : fl_lib/Electrical/Electrical Elements/Electrical Reference
  Gain : Gain  Gain=5
  Simulink-PS Converter : nesl_utility/Simulink-PS Converter  PhysicalDomain=network_engine_domain  SubClassName=ps_input  LeftPortType=input  RightPortType=output  PseudoPeriodic=off  Frequencies=[]  NoiseDistribution=none  NoiseParameters=[]  Unit=1  AffineConversion=off  FilteringAndDerivatives=provide  SimscapeFilterOrder=1  InputFilterTimeConstant=0.001  UdotUserProvided=0
  Q : PMIOPort  Side=Right
  StoredVal : Outport
  wires:
  AND/1 -> Delay One Step/1
  Store/1 -> D Latch/2
  Gain/1 -> Simulink-PS Converter/1
  D Latch/1 -> StoredVal/1, AND/1
  Cast To Double/1 -> Gain/1
  Enable/1 -> AND/2
  Data/1 -> D Latch/1
  Delay One Step/1 -> Cast To Double/1
  connections:
  Controlled Voltage Source/RConn1 -- Simulink-PS Converter/RConn1
  Electrical Reference/LConn1 -- Controlled Voltage Source/RConn2
  Controlled Voltage Source/LConn1 -- Q/RConn1

== system RAM_Design/Subsystem1/8Bit RAM 8/Subsystem10 ==
  Enable : Inport
  Data : Inport  Port=2
  Store : Inport  Port=3
  AND : Logic  IconShape=distinctive  AllPortsSameDT=off  OutDataTypeStr=boolean
  Cast To Double : DataTypeConversion  OutDataTypeStr=double  SaturateOnIntegerOverflow=off  RndMeth=Floor
  Controlled Voltage Source : fl_lib/Electrical/Electrical Sources/Controlled Voltage Source
  D Latch : simulink_extras/Flip Flops/D Latch
  Delay One Step : Delay  DelayLength=1
  Electrical Reference : fl_lib/Electrical/Electrical Elements/Electrical Reference
  Gain : Gain  Gain=5
  Simulink-PS Converter : nesl_utility/Simulink-PS Converter  PhysicalDomain=network_engine_domain  SubClassName=ps_input  LeftPortType=input  RightPortType=output  PseudoPeriodic=off  Frequencies=[]  NoiseDistribution=none  NoiseParameters=[]  Unit=1  AffineConversion=off  FilteringAndDerivatives=provide  SimscapeFilterOrder=1  InputFilterTimeConstant=0.001  UdotUserProvided=0
  Q : PMIOPort  Side=Right
  StoredVal : Outport
  wires:
  AND/1 -> Delay One Step/1
  Store/1 -> D Latch/2
  Gain/1 -> Simulink-PS Converter/1
  D Latch/1 -> StoredVal/1, AND/1
  Cast To Double/1 -> Gain/1
  Enable/1 -> AND/2
  Data/1 -> D Latch/1
  Delay One Step/1 -> Cast To Double/1
  connections:
  Controlled Voltage Source/RConn1 -- Simulink-PS Converter/RConn1
  Electrical Reference/LConn1 -- Controlled Voltage Source/RConn2
  Controlled Voltage Source/LConn1 -- Q/RConn1

== system RAM_Design/Subsystem1/8Bit RAM 8/Subsystem11 ==
  Enable : Inport
  Data : Inport  Port=2
  Store : Inport  Port=3
  AND : Logic  IconShape=distinctive  AllPortsSameDT=off  OutDataTypeStr=boolean
  Cast To Double : DataTypeConversion  OutDataTypeStr=double  SaturateOnIntegerOverflow=off  RndMeth=Floor
  Controlled Voltage Source : fl_lib/Electrical/Electrical Sources/Controlled Voltage Source
  D Latch : simulink_extras/Flip Flops/D Latch
  Delay One Step : Delay  DelayLength=1
  Electrical Reference : fl_lib/Electrical/Electrical Elements/Electrical Reference
  Gain : Gain  Gain=5
  Simulink-PS Converter : nesl_utility/Simulink-PS Converter  PhysicalDomain=network_engine_domain  SubClassName=ps_input  LeftPortType=input  RightPortType=output  PseudoPeriodic=off  Frequencies=[]  NoiseDistribution=none  NoiseParameters=[]  Unit=1  AffineConversion=off  FilteringAndDerivatives=provide  SimscapeFilterOrder=1  InputFilterTimeConstant=0.001  UdotUserProvided=0
  Q : PMIOPort  Side=Right
  StoredVal : Outport
  wires:
  AND/1 -> Delay One Step/1
  Store/1 -> D Latch/2
  Gain/1 -> Simulink-PS Converter/1
  D Latch/1 -> StoredVal/1, AND/1
  Cast To Double/1 -> Gain/1
  Enable/1 -> AND/2
  Data/1 -> D Latch/1
  Delay One Step/1 -> Cast To Double/1
  connections:
  Controlled Voltage Source/RConn1 -- Simulink-PS Converter/RConn1
  Electrical Reference/LConn1 -- Controlled Voltage Source/RConn2
  Controlled Voltage Source/LConn1 -- Q/RConn1

== system RAM_Design/Subsystem1/8Bit RAM 8/Subsystem12 ==
  Enable : Inport
  Data : Inport  Port=2
  Store : Inport  Port=3
  AND : Logic  IconShape=distinctive  AllPortsSameDT=off  OutDataTypeStr=boolean
  Cast To Double : DataTypeConversion  OutDataTypeStr=double  SaturateOnIntegerOverflow=off  RndMeth=Floor
  Controlled Voltage Source : fl_lib/Electrical/Electrical Sources/Controlled Voltage Source
  D Latch : simulink_extras/Flip Flops/D Latch
  Delay One Step : Delay  DelayLength=1
  Electrical Reference : fl_lib/Electrical/Electrical Elements/Electrical Reference
  Gain : Gain  Gain=5
  Simulink-PS Converter : nesl_utility/Simulink-PS Converter  PhysicalDomain=network_engine_domain  SubClassName=ps_input  LeftPortType=input  RightPortType=output  PseudoPeriodic=off  Frequencies=[]  NoiseDistribution=none  NoiseParameters=[]  Unit=1  AffineConversion=off  FilteringAndDerivatives=provide  SimscapeFilterOrder=1  InputFilterTimeConstant=0.001  UdotUserProvided=0
  Q : PMIOPort  Side=Right
  StoredVal : Outport
  wires:
  AND/1 -> Delay One Step/1
  Store/1 -> D Latch/2
  Gain/1 -> Simulink-PS Converter/1
  D Latch/1 -> StoredVal/1, AND/1
  Cast To Double/1 -> Gain/1
  Enable/1 -> AND/2
  Data/1 -> D Latch/1
  Delay One Step/1 -> Cast To Double/1
  connections:
  Controlled Voltage Source/RConn1 -- Simulink-PS Converter/RConn1
  Electrical Reference/LConn1 -- Controlled Voltage Source/RConn2
  Controlled Voltage Source/LConn1 -- Q/RConn1

== system RAM_Design/Subsystem1/8Bit RAM 8/Subsystem13 ==
  Enable : Inport
  Data : Inport  Port=2
  Store : Inport  Port=3
  AND : Logic  IconShape=distinctive  AllPortsSameDT=off  OutDataTypeStr=boolean
  Cast To Double : DataTypeConversion  OutDataTypeStr=double  SaturateOnIntegerOverflow=off  RndMeth=Floor
  Controlled Voltage Source : fl_lib/Electrical/Electrical Sources/Controlled Voltage Source
  D Latch : simulink_extras/Flip Flops/D Latch
  Delay One Step : Delay  DelayLength=1
  Electrical Reference : fl_lib/Electrical/Electrical Elements/Electrical Reference
  Gain : Gain  Gain=5
  Simulink-PS Converter : nesl_utility/Simulink-PS Converter  PhysicalDomain=network_engine_domain  SubClassName=ps_input  LeftPortType=input  RightPortType=output  PseudoPeriodic=off  Frequencies=[]  NoiseDistribution=none  NoiseParameters=[]  Unit=1  AffineConversion=off  FilteringAndDerivatives=provide  SimscapeFilterOrder=1  InputFilterTimeConstant=0.001  UdotUserProvided=0
  Q : PMIOPort  Side=Right
  StoredVal : Outport
  wires:
  AND/1 -> Delay One Step/1
  Store/1 -> D Latch/2
  Gain/1 -> Simulink-PS Converter/1
  D Latch/1 -> StoredVal/1, AND/1
  Cast To Double/1 -> Gain/1
  Enable/1 -> AND/2
  Data/1 -> D Latch/1
  Delay One Step/1 -> Cast To Double/1
  connections:
  Controlled Voltage Source/RConn1 -- Simulink-PS Converter/RConn1
  Electrical Reference/LConn1 -- Controlled Voltage Source/RConn2
  Controlled Voltage Source/LConn1 -- Q/RConn1

== system RAM_Design/Subsystem1/8Bit RAM 8/Subsystem14 ==
  Enable : Inport
  Data : Inport  Port=2
  Store : Inport  Port=3
  AND : Logic  IconShape=distinctive  AllPortsSameDT=off  OutDataTypeStr=boolean
  Cast To Double : DataTypeConversion  OutDataTypeStr=double  SaturateOnIntegerOverflow=off  RndMeth=Floor
  Controlled Voltage Source : fl_lib/Electrical/Electrical Sources/Controlled Voltage Source
  D Latch : simulink_extras/Flip Flops/D Latch
  Delay One Step : Delay  DelayLength=1
  Electrical Reference : fl_lib/Electrical/Electrical Elements/Electrical Reference
  Gain : Gain  Gain=5
  Simulink-PS Converter : nesl_utility/Simulink-PS Converter  PhysicalDomain=network_engine_domain  SubClassName=ps_input  LeftPortType=input  RightPortType=output  PseudoPeriodic=off  Frequencies=[]  NoiseDistribution=none  NoiseParameters=[]  Unit=1  AffineConversion=off  FilteringAndDerivatives=provide  SimscapeFilterOrder=1  InputFilterTimeConstant=0.001  UdotUserProvided=0
  Q : PMIOPort  Side=Right
  StoredVal : Outport
  wires:
  AND/1 -> Delay One Step/1
  Store/1 -> D Latch/2
  Gain/1 -> Simulink-PS Converter/1
  D Latch/1 -> StoredVal/1, AND/1
  Cast To Double/1 -> Gain/1
  Enable/1 -> AND/2
  Data/1 -> D Latch/1
  Delay One Step/1 -> Cast To Double/1
  connections:
  Controlled Voltage Source/RConn1 -- Simulink-PS Converter/RConn1
  Electrical Reference/LConn1 -- Controlled Voltage Source/RConn2
  Controlled Voltage Source/LConn1 -- Q/RConn1

== system RAM_Design/Subsystem1/8Bit RAM 8/Subsystem15 ==
  Enable : Inport
  Data : Inport  Port=2
  Store : Inport  Port=3
  AND : Logic  IconShape=distinctive  AllPortsSameDT=off  OutDataTypeStr=boolean
  Cast To Double : DataTypeConversion  OutDataTypeStr=double  SaturateOnIntegerOverflow=off  RndMeth=Floor
  Controlled Voltage Source : fl_lib/Electrical/Electrical Sources/Controlled Voltage Source
  D Latch : simulink_extras/Flip Flops/D Latch
  Delay One Step : Delay  DelayLength=1
  Electrical Reference : fl_lib/Electrical/Electrical Elements/Electrical Reference
  Gain : Gain  Gain=5
  Simulink-PS Converter : nesl_utility/Simulink-PS Converter  PhysicalDomain=network_engine_domain  SubClassName=ps_input  LeftPortType=input  RightPortType=output  PseudoPeriodic=off  Frequencies=[]  NoiseDistribution=none  NoiseParameters=[]  Unit=1  AffineConversion=off  FilteringAndDerivatives=provide  SimscapeFilterOrder=1  InputFilterTimeConstant=0.001  UdotUserProvided=0
  Q : PMIOPort  Side=Right
  StoredVal : Outport
  wires:
  AND/1 -> Delay One Step/1
  Store/1 -> D Latch/2
  Gain/1 -> Simulink-PS Converter/1
  D Latch/1 -> StoredVal/1, AND/1
  Cast To Double/1 -> Gain/1
  Enable/1 -> AND/2
  Data/1 -> D Latch/1
  Delay One Step/1 -> Cast To Double/1
  connections:
  Controlled Voltage Source/RConn1 -- Simulink-PS Converter/RConn1
  Electrical Reference/LConn1 -- Controlled Voltage Source/RConn2
  Controlled Voltage Source/LConn1 -- Q/RConn1

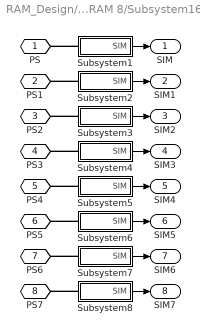
== system RAM_Design/Subsystem1/8Bit RAM 8/Subsystem16 ==
  Subsystem1 : Subsystem
  Subsystem2 : Subsystem
  Subsystem3 : Subsystem
  Subsystem4 : Subsystem
  Subsystem5 : Subsystem
  Subsystem6 : Subsystem
  Subsystem7 : Subsystem
  Subsystem8 : Subsystem
  PS : PMIOPort  Side=Left
  PS1 : PMIOPort  Port=2  Side=Left
  PS2 : PMIOPort  Port=3  Side=Left
  PS3 : PMIOPort  Port=4  Side=Left
  PS4 : PMIOPort  Port=5  Side=Left
  PS5 : PMIOPort  Port=6  Side=Left
  PS6 : PMIOPort  Port=7  Side=Left
  PS7 : PMIOPort  Port=8  Side=Left
  SIM : Outport
  SIM1 : Outport  Port=2
  SIM2 : Outport  Port=3
  SIM3 : Outport  Port=4
  SIM4 : Outport  Port=5
  SIM5 : Outport  Port=6
  SIM6 : Outport  Port=7
  SIM7 : Outport  Port=8
  wires:
  Subsystem7/1(SIM) -> SIM6/1
  Subsystem8/1(SIM) -> SIM7/1
  Subsystem3/1(SIM) -> SIM2/1
  Subsystem4/1(SIM) -> SIM3/1
  Subsystem6/1(SIM) -> SIM5/1
  Subsystem2/1(SIM) -> SIM1/1
  Subsystem5/1(SIM) -> SIM4/1
  Subsystem1/1(SIM) -> SIM/1
  connections:
  Subsystem1/LConn1 -- PS/RConn1
  Subsystem8/LConn1 -- PS7/RConn1
  Subsystem5/LConn1 -- PS4/RConn1
  Subsystem6/LConn1 -- PS5/RConn1
  Subsystem7/LConn1 -- PS6/RConn1
  Subsystem3/LConn1 -- PS2/RConn1
  Subsystem4/LConn1 -- PS3/RConn1
  Subsystem2/LConn1 -- PS1/RConn1

== system RAM_Design/Subsystem1/8Bit RAM 8/Subsystem2 ==
  Cast To Boolean : DataTypeConversion  OutDataTypeStr=boolean  SaturateOnIntegerOverflow=off  RndMeth=Floor
  Delay One Step : Delay  DelayLength=1
  Electrical Reference : fl_lib/Electrical/Electrical Elements/Electrical Reference
  Gain : Gain  Gain=0.2
  PS-Simulink Converter : nesl_utility/PS-Simulink Converter  PhysicalDomain=network_engine_domain  SubClassName=ps_output  LeftPortType=input  RightPortType=output  PseudoPeriodic=off  Frequencies=[]  VectorFormat=inherit  Unit=inherit  AffineConversion=off
  Voltage Sensor : fl_lib/Electrical/Electrical Sensors/Voltage Sensor
  PS : PMIOPort  Side=Left
  SIM : Outport
  wires:
  PS-Simulink Converter/1 -> Gain/1
  Cast To Boolean/1 -> Delay One Step/1
  Gain/1 -> Cast To Boolean/1
  Delay One Step/1 -> SIM/1
  connections:
  PS/RConn1 -- Voltage Sensor/LConn1
  Electrical Reference/LConn1 -- Voltage Sensor/RConn2
  PS-Simulink Converter/LConn1 -- Voltage Sensor/RConn1

== system RAM_Design/Subsystem1/8Bit RAM 8/Subsystem3 ==
  Cast To Boolean : DataTypeConversion  OutDataTypeStr=boolean  SaturateOnIntegerOverflow=off  RndMeth=Floor
  Delay One Step : Delay  DelayLength=1
  Electrical Reference : fl_lib/Electrical/Electrical Elements/Electrical Reference
  Gain : Gain  Gain=0.2
  PS-Simulink Converter : nesl_utility/PS-Simulink Converter  PhysicalDomain=network_engine_domain  SubClassName=ps_output  LeftPortType=input  RightPortType=output  PseudoPeriodic=off  Frequencies=[]  VectorFormat=inherit  Unit=inherit  AffineConversion=off
  Voltage Sensor : fl_lib/Electrical/Electrical Sensors/Voltage Sensor
  PS : PMIOPort  Side=Left
  SIM : Outport
  wires:
  PS-Simulink Converter/1 -> Gain/1
  Cast To Boolean/1 -> Delay One Step/1
  Gain/1 -> Cast To Boolean/1
  Delay One Step/1 -> SIM/1
  connections:
  PS/RConn1 -- Voltage Sensor/LConn1
  Electrical Reference/LConn1 -- Voltage Sensor/RConn2
  PS-Simulink Converter/LConn1 -- Voltage Sensor/RConn1
